simulink model "tutorial41_callbacks"  (R2025a)
settings: Solver=VariableStepAuto  StartTime=0.0  StopTime=10.0  RelTol=1e-3
PreLoadFcn:
  | disp('   [PreLoadFcn] 正在加载参数...');
InitFcn:
  | fprintf('   [InitFcn] 参数检查通过: Kp=%.1f, Ki=%.1f\n', Kp, Ki);
  | fprintf('   [InitFcn] 时间: %s\n', datestr(now));
  | last_sim_time = now;
StopFcn:
  | disp('   [StopFcn] 仿真结束, 自动保存结果...');
  | try
  |     sim_data.t = tout;
  |     sim_data.y = yout;
  |     save('C:\\Users\\xing2\\Desktop\\Simulink\\models\\tutorial41_results.mat', 'sim_data');
  |     disp('   [StopFcn] 结果已保存');
  | catch ME
  |     disp(['   [StopFcn] 保存失败: ' ME.message]);
  | end
undefined symbols (not defined in the file): Ki, Kp
settings Model: Creator=xing2  LastModifiedBy=xing2

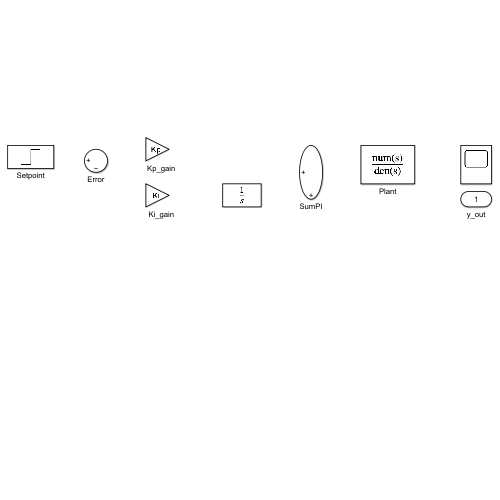
[thumbnail: Simulink's stored preview of the top-level diagram]
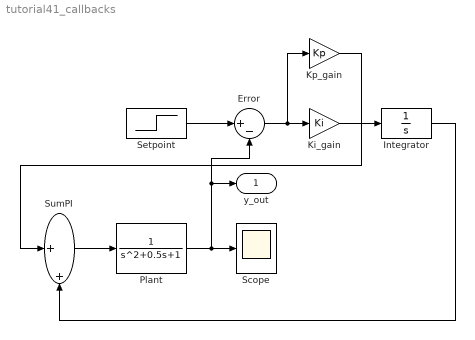
== system tutorial41_callbacks ==
  Error : Sum  Inputs=|+-
  Integrator : Integrator
  Ki_gain : Gain  Gain=Ki
  Kp_gain : Gain  Gain=Kp
  Plant : TransferFcn  Denominator=[1 0.5 1]
  Scope : Scope
  Setpoint : Step  Time=0.5  SampleTime=0
  SumPI : Sum  Inputs=|++
  y_out : Outport
  wires:
  Plant/1 -> Error/2, y_out/1, Scope/1
  SumPI/1 -> Plant/1
  Setpoint/1 -> Error/1
  Ki_gain/1 -> Integrator/1
  Kp_gain/1 -> SumPI/1
  Error/1 -> Kp_gain/1, Ki_gain/1
  Integrator/1 -> SumPI/2
